simulink model "state_space_all_reduce_uio"  (R2018a)
settings: Solver=FixedStepAuto  StartTime=0.0  StopTime=3  FixedStep=tm  MaxStep=1e-4  RelTol=1e-5  AbsTol=1e-5
InitFcn:
  | SimulinkInit_linea_transmision
values from neighbouring files (symbols this model uses):
  b = 4.91    [SimulinkInit_linea_transmision.m]
  C = 1    [SimulinkInit_linea_transmision.m]
  C1 = 22e-6    (= 2.2e-05)    [SimulinkInit_linea_transmision.m]
  C2 = 22e-6    (= 2.2e-05)    [SimulinkInit_linea_transmision.m]
  C3 = 610e-6    (= 0.00061)    [SimulinkInit_linea_transmision.m]
  Cl = 20000e-6    (= 0.02)    [SimulinkInit_linea_transmision.m]
  Jd = 0.3    [SimulinkInit_linea_transmision.m]
  K = 25    [SimulinkInit_linea_transmision.m]    (also in uio_linear.m = K1+E*H)
  K1 = 9.66    [SimulinkInit_linea_transmision.m]    (also in uio_linear.m = K1')
  K11 = 0.8    [SimulinkInit_linea_transmision.m]
  K1d = 1.15    [SimulinkInit_linea_transmision.m]
  K2 = 6.97    [SimulinkInit_linea_transmision.m]
  K22 = 0.2    [SimulinkInit_linea_transmision.m]
  K2d = 1    [SimulinkInit_linea_transmision.m]
  K3 = 31.8    [SimulinkInit_linea_transmision.m]
  K33 = 0.23    [SimulinkInit_linea_transmision.m]
  K3d = 1    [SimulinkInit_linea_transmision.m]
  K4 = 15.1    [SimulinkInit_linea_transmision.m]
  Kd = 0.02    [SimulinkInit_linea_transmision.m]
  Kdc = 0.02    [SimulinkInit_linea_transmision.m]
  Kf = 1    [SimulinkInit_linea_transmision.m]
  Kh = 1.2    [SimulinkInit_linea_transmision.m]
  Ks = 21.5    [SimulinkInit_linea_transmision.m]
  Ksc = 3    [SimulinkInit_linea_transmision.m]
  Kv = 1    [SimulinkInit_linea_transmision.m]
  L = 5.2    [SimulinkInit_linea_transmision.m]
  L1 = 40e-3    (= 0.04)    [SimulinkInit_linea_transmision.m]
  L2 = 30e-3    (= 0.03)    [SimulinkInit_linea_transmision.m]
  L3 = 5e-3    (= 0.005)    [SimulinkInit_linea_transmision.m]
  L4 = 35e-6    (= 3.5e-05)    [SimulinkInit_linea_transmision.m]
  L5 = 22e-6    (= 2.2e-05)    [SimulinkInit_linea_transmision.m]
  L6 = 10e-6    (= 1e-05)    [SimulinkInit_linea_transmision.m]
  Pd = 0.1    [SimulinkInit_linea_transmision.m]
  R = 10    [SimulinkInit_linea_transmision.m]
  R1 = 0.1    [SimulinkInit_linea_transmision.m]
  R2 = 0.2    [SimulinkInit_linea_transmision.m]
  R3 = 1e-3    (= 0.001)    [SimulinkInit_linea_transmision.m]
  R4 = 0.005    [SimulinkInit_linea_transmision.m]
  R5 = 0.0012    [SimulinkInit_linea_transmision.m]
  R6 = 0.001    [SimulinkInit_linea_transmision.m]
  RL = 10    [SimulinkInit_linea_transmision.m]
  Sbin = 13.8    [SimulinkInit_linea_transmision.m]
  Svin = 2.91    [SimulinkInit_linea_transmision.m]
  T1 = 0.4    [SimulinkInit_linea_transmision.m]
  T2 = 1    [SimulinkInit_linea_transmision.m]
  T3 = 15    [SimulinkInit_linea_transmision.m]
  T4 = 2.5    [SimulinkInit_linea_transmision.m]
  Tao1d = 0.5    [SimulinkInit_linea_transmision.m]
  Tao2d = 0.125    [SimulinkInit_linea_transmision.m]
  Tcd = 0.2    [SimulinkInit_linea_transmision.m]
  Tcr = 0.01    [SimulinkInit_linea_transmision.m]
  Tf = 0.04    [SimulinkInit_linea_transmision.m]
  Tr = 950    [SimulinkInit_linea_transmision.m]
  Tt = 450    [SimulinkInit_linea_transmision.m]
  Ttd = 0.04    [SimulinkInit_linea_transmision.m]
  Tv = 0.05    [SimulinkInit_linea_transmision.m]
  V = 20    [SimulinkInit_linea_transmision.m]
  wref = 70000    [SimulinkInit_linea_transmision.m]
  X_acid = 1.2    [SimulinkInit_linea_transmision.m]
  X_meth = 0.35    [SimulinkInit_linea_transmision.m]
  Z = 3    [SimulinkInit_linea_transmision.m]
undefined symbols (not defined in the file or in its folder): Ad, ataque, Bd, c11, c12, c13, c14, C1o, c21, c22, c23, c24, C2o, c31, c32, c33, c34, C3o, c41, c42, c43, c44, C4o, Cd, F1, F2, F3, F4, H1, H2, H3, H4, K1U, K2U, K3U, K4U, T1s, T2s, T3s, T4s, T5s, tao1, tao2, taod, tm, uio1r, uio2r, uio3r, uio4r
libraries: neural x277, dsparch4 x4, powerlib_meascontrol x4, mpclib x1, simulink x1
(part 1 of 16)
settings Model: Creator=MarioAndres  LastModifiedBy=carma

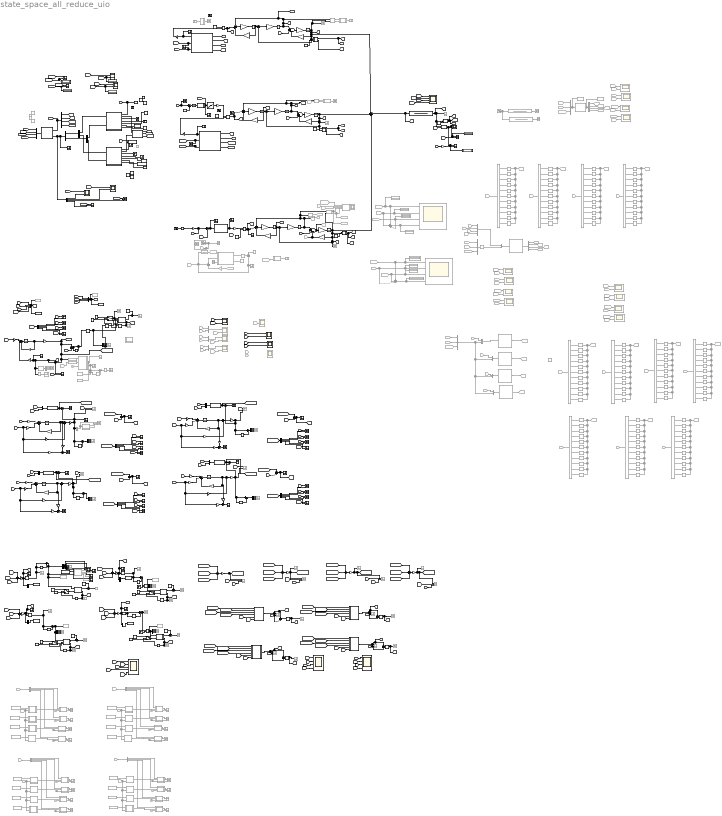
== system state_space_all_reduce_uio ==
  note: Nodo De Optimizacion
  note: CSI1-Biomasa
  note: CSI2-pv
  note: VSI-Diesel
  note: Carga RLC
  note: Attack Detection
  note: Attack Isolation I2
  note: Attack Isolation I3
  note: Attack Isolation I1
  note: Attack Isolation Vsi
  note: Alarm I1
  note: Alarm I3
  note: Alarm I2
  note: Alarm V
  note: Attack Quantification
  1-D Lookup Table2 : Lookup_n-D  NumberOfTableDimensions=1  BreakpointsForDimension1=[0 10 20 30 40 50 70 80 100]  Table=[0 10 200 500 800 1000 1140 1150 1200]  InternalRulePriority=Speed  RndMeth=Simplest  InputSameDT=on
  Abs{,1..3,5..9} (9 alike) : Abs
  Abs4 : Abs  Commented=on
  CSI_Control_BIO : Subsystem  mask{A=[0.0201   -0.039932     0.01986], B=[1     -1.9966       0.998], T=0.0001, st_time=0, Dn=[1     -1.0364], Dd=[1    -0.96364]}
      mask prompts: A "Numerador del control PR(z)"; B "Denominador del control PR(z)"; T "Tiempo de muestreo"; st_time "Tiempo_muerto"; Dn "Dn (Numerador de D(z))"; Dd "Dd (numerador de D(z))"
      mask DialogControl descripcion Prompt: Lazo de control de corriente para inversor monofasico. La entrada es un setpoint de potencia [P, Q]. Con ese setpoint se calcula la referencia de corriente sinusoidal deacuerdo a la tension medida de la red. Por lo anterior este controlador solo es valido para un inversor conectado a la red pues hara que se comporte como un CSI.
      mask DialogControl Control2 Prompt: Dn y Dd corresponden al numerador y denominador de la funcion de transferencia en Z (denominada D(z)) que hara un desfase de 90 de las señales medidas de tension y corriente del inversor. Estos desfases permiten mimificar las señales alfa y beta, de esta forma usar la misma teoria de potencia instantanea para el caso monofasico.
  CSI_Control_BIO1 : Subsystem  mask{A=[0.0201   -0.039932     0.01986], B=[1     -1.9966       0.998], T=0.0001, st_time=0, Dn=[1     -1.0364], Dd=[1    -0.96364]}
      mask prompts: A "Numerador del control PR(z)"; B "Denominador del control PR(z)"; T "Tiempo de muestreo"; st_time "Tiempo_muerto"; Dn "Dn (Numerador de D(z))"; Dd "Dd (numerador de D(z))"
      mask DialogControl descripcion Prompt: Lazo de control de corriente para inversor monofasico. La entrada es un setpoint de potencia [P, Q]. Con ese setpoint se calcula la referencia de corriente sinusoidal deacuerdo a la tension medida de la red. Por lo anterior este controlador solo es valido para un inversor conectado a la red pues hara que se comporte como un CSI.
      mask DialogControl Control2 Prompt: Dn y Dd corresponden al numerador y denominador de la funcion de transferencia en Z (denominada D(z)) que hara un desfase de 90 de las señales medidas de tension y corriente del inversor. Estos desfases permiten mimificar las señales alfa y beta, de esta forma usar la misma teoria de potencia instantanea para el caso monofasico.
  Clock : Clock
  Clock{1,4..19} (17 alike) : Clock  Commented=on
  Clock2 : Clock
  Constant : Constant  Commented=on  Value=-400
  Constant1 : Constant  Commented=on  Value=5000
  Constant{5..6,9..10,12,22..23,27..28,32} (10 alike) : Constant
  Constant{4,11,14,18,20,25} (6 alike) : Constant  Value=1000
  Constant13 : Constant  Value=500
  Constant15 : Constant  Value=1528
  Constant16 : Constant  Value=1200
  Constant17 : Constant  Value=115400
  Constant19 : Constant  Value=800
  Constant2 : Constant  Commented=on  Value=5000
  Constant{7..8,21,24,31} (5 alike) : Constant  Value=0
  Constant26 : Constant  Commented=on  Value=11210
  Constant29 : Constant  Commented=on  Value=1000
  Constant3 : Constant  Commented=on  Value=8000
  Constant30 : Constant  Commented=on  Value=0.1
  Constant{33..36} (4 alike) : Constant  Value=ataque
  Constant37 : Constant  Value=[c11 c12 c13 c14]
  Constant38 : Constant  Commented=on  Value=[c11 c11 c11]
  Constant39 : Constant  Commented=on  Value=[c12 c12 c12]
  Constant40 : Constant  Commented=on  Value=[c13 c13 c13]
  Constant41 : Constant  Commented=on  Value=[c14 c14 c14]
  Constant42 : Constant  Commented=on  Value=[c21 c21 c21]
  Constant43 : Constant  Commented=on  Value=[c22 c22 c22]
  Constant44 : Constant  Commented=on  Value=[c23 c23 c23]
  Constant45 : Constant  Commented=on  Value=[c24 c24 c24]
  Constant46 : Constant  Commented=on  Value=[c31 c31 c31]
  Constant47 : Constant  Commented=on  Value=[c32 c32 c32]
  Constant48 : Constant  Commented=on  Value=[c33 c33 c33]
  Constant49 : Constant  Commented=on  Value=[c34 c34 c34]
  Constant50 : Constant  Commented=on  Value=[c41 c41 c41]
  Constant51 : Constant  Commented=on  Value=[c42 c42 c42]
  Constant52 : Constant  Commented=on  Value=[c43 c43 c43]
  Constant53 : Constant  Commented=on  Value=[c44 c44 c44]  VectorParams1D=off
  Control PR VSI1 : Subsystem
  Current Panel : Constant  Value=1.5
  Delay : Delay  DelayLength=1
  Delay{1..2,16,30,34} (5 alike) : Delay  Commented=on  DelayLength=11
  Delay{10,13,24,27} (4 alike) : Delay  Commented=on  DelayLength=3
  Delay{57,71,85,90,100..101,112} (7 alike) : Delay  Commented=on  DelayLength=8  SampleTime=2*tm
  Delay{46..47,58,62,72,102,113} (7 alike) : Delay  Commented=on  DelayLength=9  SampleTime=2*tm
  Delay{48,59,63,74,91,103,114} (7 alike) : Delay  Commented=on  DelayLength=10  SampleTime=2*tm
  Delay{49,60,64,75,92,104,115} (7 alike) : Delay  Commented=on  DelayLength=11  SampleTime=2*tm
  Delay{50,61,73,76,93,105,116} (7 alike) : Delay  Commented=on  DelayLength=1  SampleTime=2*tm
  Delay{51,65,77..78,94,106,117} (7 alike) : Delay  Commented=on  SampleTime=2*tm
  Delay{52,66,79..80,95,107,118} (7 alike) : Delay  Commented=on  DelayLength=3  SampleTime=2*tm
  Delay{53,67,81,86,96,108,119} (7 alike) : Delay  Commented=on  DelayLength=4  SampleTime=2*tm
  Delay{54,68,82,87,97,109,120} (7 alike) : Delay  Commented=on  DelayLength=5  SampleTime=2*tm
  Delay{11,14,25,28} (4 alike) : Delay  Commented=on
  Delay{55,69,83,88,98,110,121} (7 alike) : Delay  Commented=on  DelayLength=6  SampleTime=2*tm
  Delay{56,70,84,89,99,111,122} (7 alike) : Delay  Commented=on  DelayLength=7  SampleTime=2*tm
  Delay{12,15,26,29} (4 alike) : Delay  Commented=on  DelayLength=1
  Delay{3,17,31,39} (4 alike) : Delay  Commented=on  DelayLength=10
  Delay{4,18,32,40} (4 alike) : Delay  Commented=on  DelayLength=9
  Delay{5,19,33,41} (4 alike) : Delay  Commented=on  DelayLength=8
  Delay{6,20,35,42} (4 alike) : Delay  Commented=on  DelayLength=7
  Delay{7,21,36,43} (4 alike) : Delay  Commented=on  DelayLength=6
  Delay{8,22,37,44} (4 alike) : Delay  Commented=on  DelayLength=5
  Delay{9,23,38,45} (4 alike) : Delay  Commented=on  DelayLength=4
  Demux{,5,7,18..22} (8 alike) : Demux  Commented=on
  Demux{1..4,6,8..17,24,26..29} (20 alike) : Demux
  Derivative1 : Derivative
  Derivative4 : Derivative  Commented=on  CoefficientInTFapproximation=0
  Diesel Generator2 : Subsystem  Commented=on
  Discrete State-Space : DiscreteStateSpace  A=uio1r.A  B=uio1r.B  C=uio1r.C  D=uio1r.D  SampleTime=tm
  Discrete State-Space1 : DiscreteStateSpace  A=uio4r.A  B=uio4r.B  C=uio4r.C  D=uio4r.D  SampleTime=tm
  Discrete State-Space2 : DiscreteStateSpace  A=uio2r.A  B=uio2r.B  C=uio2r.C  D=uio2r.D  SampleTime=tm
  Discrete State-Space3 : DiscreteStateSpace  A=uio3r.A  B=uio3r.B  C=uio3r.C  D=uio3r.D  SampleTime=tm
  Display{,1..3,6..9} (8 alike) : Display  Commented=on
      Display settings: Decimation=6
      Display1 settings: Decimation=3
      Display2 settings: Decimation=3
      Display3 settings: Decimation=6
      Display6 settings: Decimation=2
      Display7 settings: Decimation=3
      Display8 settings: Decimation=3
      Display9 settings: Decimation=2
  Display{4..5,10..13} (6 alike) : Display
      Display10 settings: Decimation=3
      Display11 settings: Decimation=3
      Display12 settings: Decimation=3
      Display13 settings: Decimation=3
      Display4 settings: Decimation=3
      Display5 settings: Decimation=2
  From : From  Commented=on  GotoTag=i1model
  From14 : From  Commented=on  GotoTag=i1
  From{15,47,184,214} (4 alike) : From  Commented=on  GotoTag=i2
  From{24,154,185,215} (4 alike) : From  Commented=on  GotoTag=Vload
  From160 : From  Commented=on  GotoTag=Qo_diesel
  From161 : From  Commented=on  GotoTag=Po_diesel2
  From162 : From  Commented=on  GotoTag=Po_diesel
  From163 : From  Commented=on  GotoTag=Po_bio
  From164 : From  Commented=on  GotoTag=Qo_bio
  From165 : From  Commented=on  GotoTag=Qo_diesel2
  From167 : From  Commented=on  GotoTag=I3
  From168 : From  Commented=on  GotoTag=I2
  From169 : From  Commented=on  GotoTag=I1
  From170 : From  Commented=on  GotoTag=I1r
  From171 : From  Commented=on  GotoTag=I2r
  From172 : From  Commented=on  GotoTag=I3r
  From174 : From  Commented=on  GotoTag=ruo1
  From176 : From  Commented=on  GotoTag=ruo3
  From177 : From  Commented=on  GotoTag=ruo2
  From181 : From  Commented=on  GotoTag=Vlreal
  From182 : From  Commented=on  GotoTag=i1model
  From183 : From  Commented=on  GotoTag=i1
  From186 : From  Commented=on  GotoTag=i3
  From187 : From  Commented=on  GotoTag=i2model
  From188 : From  Commented=on  GotoTag=i3model
  From189 : From  Commented=on  GotoTag=Vloadm
  From190 : From  Commented=on  GotoTag=u2
  From191 : From  Commented=on  GotoTag=u3
  From192 : From  Commented=on  GotoTag=u1
  From193 : From  Commented=on  GotoTag=i1model
  From194 : From  Commented=on  GotoTag=i2model
  From195 : From  Commented=on  GotoTag=i3model
  From196 : From  Commented=on  GotoTag=Vloadm
  From197 : From  Commented=on  GotoTag=i1nn
  From198 : From  Commented=on  GotoTag=i2nn
  From199 : From  Commented=on  GotoTag=i3nn
  From200 : From  Commented=on  GotoTag=vnn
  From201 : From  Commented=on  GotoTag=u2nn
  From202 : From  Commented=on  GotoTag=u3nn
  From203 : From  Commented=on  GotoTag=u1nn
  From204 : From  Commented=on  GotoTag=i1model1
  From205 : From  Commented=on  GotoTag=i2model1
  From206 : From  Commented=on  GotoTag=i3model1
  From207 : From  Commented=on  GotoTag=Vloadm1
  From208 : From  Commented=on  GotoTag=i1nn1
  From209 : From  Commented=on  GotoTag=i2nn1
  From210 : From  Commented=on  GotoTag=i3nn1
  From211 : From  Commented=on  GotoTag=vnn1
  From212 : From  Commented=on  GotoTag=i1model1
  From213 : From  Commented=on  GotoTag=i1
  From216 : From  Commented=on  GotoTag=i3
  From217 : From  Commented=on  GotoTag=i2model1
  From218 : From  Commented=on  GotoTag=i3model1
  From219 : From  Commented=on  GotoTag=Vloadm1
  From220 : From  Commented=on  GotoTag=u1
  From221 : From  Commented=on  GotoTag=u2
  From222 : From  Commented=on  GotoTag=u3
  From{224,226,228,230} (4 alike) : From  Commented=on  GotoTag=u_fs
  From225 : From  Commented=on  GotoTag=uio1
  From227 : From  Commented=on  GotoTag=uio2
  From229 : From  Commented=on  GotoTag=uio3
  From231 : From  Commented=on  GotoTag=uio4
  From25 : From  Commented=on  GotoTag=i3
  From264 : From  Commented=on  GotoTag=I3
  From269 : From  Commented=on  GotoTag=I3r
  From30 : From  Commented=on  GotoTag=u2
  From33 : From  Commented=on  GotoTag=u3
  From37 : From  Commented=on  GotoTag=Papadiel
  From38 : From  Commented=on  GotoTag=Paparente
  From39 : From  Commented=on  GotoTag=Q_ref
  From40 : From  Commented=on  GotoTag=P_ref
  From41 : From  Commented=on  GotoTag=Io_diesel
  From6 : From  Commented=on  GotoTag=i2model
  From60 : From  Commented=on  GotoTag=y_ma
  From7 : From  Commented=on  GotoTag=i3model
  From8 : From  Commented=on  GotoTag=Vloadm
  From9 : From  Commented=on  GotoTag=u1
  Function Fitting Neural Network : Subsystem  Commented=on
      mask help: Function Fitting Neural Network
      mask Display: e = 0.06;c1 = [120 150 230]/255;c2 = ([120 150 230]+0)/383;c3 = ([120 150 230]+128)/383;patch([0 1 1 0],[0 0 1 1],c1);patch([0 1 1 1-e 1-e 0+e],[0 0 1 1-e 0+e 0+e],c2);patch([0 0 1 1-e 0+e 0+e],[0 1 1 1-e 1-e 0+e],c3);plot([0 1 1 0 0],[0 0 1 1 0]);fprintf('NNET');port_label('input',1,' Input');port_label('output',1,'Output ');
  Function Fitting Neural Network1 : Subsystem  Commented=on
      mask help: Function Fitting Neural Network
      mask Display: e = 0.06;c1 = [120 150 230]/255;c2 = ([120 150 230]+0)/383;c3 = ([120 150 230]+128)/383;patch([0 1 1 0],[0 0 1 1],c1);patch([0 1 1 1-e 1-e 0+e],[0 0 1 1-e 0+e 0+e],c2);patch([0 0 1 1-e 0+e 0+e],[0 1 1 1-e 1-e 0+e],c3);plot([0 1 1 0 0],[0 0 1 1 0]);fprintf('NNET');port_label('input',1,' Input');port_label('output',1,'Output ');
  Function Fitting Neural Network2 : Subsystem  Commented=on
      mask help: Function Fitting Neural Network
      mask Display: e = 0.06;c1 = [120 150 230]/255;c2 = ([120 150 230]+0)/383;c3 = ([120 150 230]+128)/383;patch([0 1 1 0],[0 0 1 1],c1);patch([0 1 1 1-e 1-e 0+e],[0 0 1 1-e 0+e 0+e],c2);patch([0 0 1 1-e 0+e 0+e],[0 1 1 1-e 1-e 0+e],c3);plot([0 1 1 0 0],[0 0 1 1 0]);fprintf('NNET');port_label('input',1,' Input');port_label('output',1,'Output ');
  Function Fitting Neural Network3 : Subsystem  Commented=on
      mask help: Function Fitting Neural Network
      mask Display: e = 0.06;c1 = [120 150 230]/255;c2 = ([120 150 230]+0)/383;c3 = ([120 150 230]+128)/383;patch([0 1 1 0],[0 0 1 1],c1);patch([0 1 1 1-e 1-e 0+e],[0 0 1 1-e 0+e 0+e],c2);patch([0 0 1 1-e 0+e 0+e],[0 1 1 1-e 1-e 0+e],c3);plot([0 1 1 0 0],[0 0 1 1 0]);fprintf('NNET');port_label('input',1,' Input');port_label('output',1,'Output ');
  Function Fitting Neural Network4 : Subsystem  Commented=on
      mask help: Function Fitting Neural Network
      mask Display: e = 0.06;c1 = [120 150 230]/255;c2 = ([120 150 230]+0)/383;c3 = ([120 150 230]+128)/383;patch([0 1 1 0],[0 0 1 1],c1);patch([0 1 1 1-e 1-e 0+e],[0 0 1 1-e 0+e 0+e],c2);patch([0 0 1 1-e 0+e 0+e],[0 1 1 1-e 1-e 0+e],c3);plot([0 1 1 0 0],[0 0 1 1 0]);fprintf('NNET');port_label('input',1,' Input');port_label('output',1,'Output ');
  Gain : Gain  Gain=1/L1
  Gain1 : Gain  Gain=1/C1
  Gain10 : Gain  Gain=1/L3
  Gain11 : Gain  Gain=1/C3
  Gain12 : Gain  Gain=1/L6
  Gain13 : Gain  Gain=R6
  Gain14 : Gain  Gain=R3
  Gain{15..18} (4 alike) : Gain  Gain=2
  Gain2 : Gain  Gain=1/L4
  Gain20 : Gain  Gain=-1
  Gain21 : Gain  Commented=on  Gain=.5
  Gain{22..29} (8 alike) : Gain  Gain=1/3
  Gain3 : Gain  Gain=R4
  Gain30 : Gain  Gain=C3
  Gain4 : Gain  Gain=R1
  Gain5 : Gain  Gain=1/L2
  Gain6 : Gain  Gain=1/C2
  Gain7 : Gain  Gain=1/L5
  Gain8 : Gain  Gain=R5
  Gain9 : Gain  Gain=R2
  Goto : Goto  Commented=on  GotoTag=i1model
  Goto15 : Goto  Commented=on  GotoTag=i2model
  Goto16 : Goto  Commented=on  GotoTag=i3model
  Goto17 : Goto  Commented=on  GotoTag=v3
  Goto18 : Goto  Commented=on  GotoTag=vl6
  Goto19 : Goto  Commented=on  GotoTag=vr6
  Goto22 : Goto  Commented=on  GotoTag=Vloadm
  Goto23 : Goto  Commented=on  GotoTag=Vdc
  Goto24 : Goto  Commented=on  GotoTag=Io_diesel
  Goto61 : Goto  Commented=on  GotoTag=V_vsi
  Goto62 : Goto  Commented=on  GotoTag=a4
  Goto74 : Goto  Commented=on  GotoTag=Qo_diesel2
  Goto75 : Goto  Commented=on  GotoTag=Po_diesel2
  Goto79 : Goto  Commented=on  GotoTag=i1model
  Goto80 : Goto  Commented=on  GotoTag=i2model
  Goto81 : Goto  Commented=on  GotoTag=i3model
  Goto82 : Goto  Commented=on  GotoTag=Vloadm
  Goto83 : Goto  Commented=on  GotoTag=i1nn
  Goto84 : Goto  Commented=on  GotoTag=i2nn
  Goto85 : Goto  Commented=on  GotoTag=i3nn
  Goto86 : Goto  Commented=on  GotoTag=vnn
  Goto87 : Goto  Commented=on  GotoTag=i1model1
  Goto88 : Goto  Commented=on  GotoTag=i2model1
  Goto89 : Goto  Commented=on  GotoTag=i3model1
  Goto90 : Goto  Commented=on  GotoTag=Vloadm1
  Goto91 : Goto  Commented=on  GotoTag=i1nn1
  Goto92 : Goto  Commented=on  GotoTag=i2nn1
  Goto93 : Goto  Commented=on  GotoTag=i3nn1
  Goto94 : Goto  Commented=on  GotoTag=vnn1
  Goto95 : Goto  Commented=on  GotoTag=u1nn
  Goto96 : Goto  Commented=on  GotoTag=u2nn
  Goto97 : Goto  Commented=on  GotoTag=u3nn
  Integrator{,1..8} (9 alike) : Integrator
  Integrator9 : Integrator  LimitOutput=on  UpperSaturationLimit=1  LowerSaturationLimit=0
  LinearProg2 : MATLAB Function  TreatAsAtomicUnit=on  SystemSampleTime=1e-3
  LinearProg3 : MATLAB Function  TreatAsAtomicUnit=on  SystemSampleTime=1e-3
  MATLAB Funcionando sin Vload conectado despues del ataque : MATLAB Function  Commented=on  TreatAsAtomicUnit=on
  MATLAB Function : MATLAB Function  Commented=on  TreatAsAtomicUnit=on
  "MATLAB Function SOC " : MATLAB Function  TreatAsAtomicUnit=on
  MATLAB Function1 : MATLAB Function  TreatAsAtomicUnit=on
  MATLAB Function10 : MATLAB Function  Commented=on  TreatAsAtomicUnit=on
  MATLAB Function11 : MATLAB Function  Commented=on  TreatAsAtomicUnit=on
  MATLAB Function12 : MATLAB Function  TreatAsAtomicUnit=on
  MATLAB Function13 : MATLAB Function  TreatAsAtomicUnit=on
  MATLAB Function14 : MATLAB Function  Commented=on  TreatAsAtomicUnit=on
  MATLAB Function15 : MATLAB Function  Commented=on  TreatAsAtomicUnit=on
  MATLAB Function16 : MATLAB Function  Commented=on  TreatAsAtomicUnit=on
  MATLAB Function17 : MATLAB Function  TreatAsAtomicUnit=on
  MATLAB Function18 : MATLAB Function  TreatAsAtomicUnit=on
  MATLAB Function19 : MATLAB Function  Commented=on  TreatAsAtomicUnit=on
  MATLAB Function2 : MATLAB Function  TreatAsAtomicUnit=on
  MATLAB Function20 : MATLAB Function  Commented=on  TreatAsAtomicUnit=on
  MATLAB Function21 : MATLAB Function  Commented=on  TreatAsAtomicUnit=on
  MATLAB Function22 : MATLAB Function  Commented=on  TreatAsAtomicUnit=on
  MATLAB Function23 : MATLAB Function  Commented=on  TreatAsAtomicUnit=on
  MATLAB Function24 : MATLAB Function  Commented=on  TreatAsAtomicUnit=on
  MATLAB Function25 : MATLAB Function  Commented=on  TreatAsAtomicUnit=on
  MATLAB Function26 : MATLAB Function  Commented=on  TreatAsAtomicUnit=on
  MATLAB Function27 : MATLAB Function  Commented=on  TreatAsAtomicUnit=on
  MATLAB Function28 : MATLAB Function  Commented=on  TreatAsAtomicUnit=on
  MATLAB Function29 : MATLAB Function  Commented=on  TreatAsAtomicUnit=on
  MATLAB Function3 : MATLAB Function  Commented=on  TreatAsAtomicUnit=on
  MATLAB Function34 : MATLAB Function  TreatAsAtomicUnit=on
  MATLAB Function36 : MATLAB Function  TreatAsAtomicUnit=on
  MATLAB Function38 : MATLAB Function  TreatAsAtomicUnit=on
  MATLAB Function39 : MATLAB Function  TreatAsAtomicUnit=on
  MATLAB Function4 : MATLAB Function  Commented=on  TreatAsAtomicUnit=on
  MATLAB Function5 : MATLAB Function  Commented=on  TreatAsAtomicUnit=on
  MATLAB Function6 : MATLAB Function  Commented=on  TreatAsAtomicUnit=on
  MATLAB Function7 : MATLAB Function  Commented=on  TreatAsAtomicUnit=on
  MATLAB Function8 : MATLAB Function  Commented=on  TreatAsAtomicUnit=on
  MPC Controller : mpclib/MPC Controller  SCDEnableBlockLinearizationSpecification=on  mpcobj=mpcobj  is_multiple=0  enable_value=0  return_u0=off  updateMPCinCallerWorkspace=on  ref_from_ws=off  ref_signal_name=[]  ref_preview=off  md_from_ws=off  md_signal_name=[]  md_preview=off  from_project=off  project_file=MPCtask.mat  md_inport=off  mv_inport=off  cost_outport=off  return_sequence=off  return_qpstatus=off  return_state=off  state_inport=off  lims_inport=off  cc_inport=off  ywt_inport=off  is_designfromscratch=0  uwt_inport=off  duwt_inport=off  rhoeps_inport=off  uref_inport=off  n_ts=0.1  n_p=100  n_mv=4  n_md=0  n_ud=0  n_mo=4  n_uo=0  BlockDataType=double  SampleTimeInherited=off  switch_inport=off
  MeasureNode_I1 : Subsystem
  MeasureNode_I2 : Subsystem
  MeasureNode_I3 : Subsystem
  MeasureNode_I4 : Subsystem
  MeasureNode_I5 : Subsystem  Commented=on
  Memory{,1..13} (14 alike) : Memory
  Memory14 : Memory  Commented=on
  Mux{,14,16..18,26..28} (8 alike) : Mux  Commented=on  Inputs=2
  Mux1 : Mux  Commented=on  Inputs=3
  Mux{9..12,19..25} (11 alike) : Mux  Commented=on  Inputs=11
  Mux13 : Mux  Commented=on
  Mux15 : Mux  Commented=on  Inputs=3
  Mux2 : Mux  Commented=on  Inputs=3
  Mux{3,5..6,29..32} (7 alike) : Mux  Inputs=2
  Mux4 : Mux
  Mux7 : Mux  Inputs=3
  Mux8 : Mux
  PID Controller2 : simulink/Continuous/PID Controller  Commented=on  Controller=PID  TimeDomain=Continuous-time  SampleTime=-1  IntegratorMethod=Forward Euler  FilterMethod=Forward Euler  Form=Parallel  UseFilter=on  ControllerParametersSource=internal  P=0.000853612192208084  I=3.94394231511782e-05  D=0.00224356290205903  N=0.155980576752107  InitialConditionSource=internal  InitialConditionForIntegrator=0  InitialConditionForFilter=0  ExternalReset=none  LimitOutput=off  UpperSaturationLimit=inf  LowerSaturationLimit=-inf  LinearizeAsGain=on  AntiWindupMode=none  Kb=1  TrackingMode=off  Kt=1  PParamMin=[]  PParamMax=[]  IParamMin=[]  IParamMax=[]  DParamMin=[]  DParamMax=[]  NParamMin=[]  NParamMax=[]  KbParamMin=[]  KbParamMax=[]  KtParamMin=[]  KtParamMax=[]  POutMin=[]  POutMax=[]  IOutMin=[]  IOutMax=[]  DOutMin=[]  DOutMax=[]  NOutMin=[]  NOutMax=[]  KbOutMin=[]  KbOutMax=[]  KtOutMin=[]  KtOutMax=[]  IntegratorOutMin=[]  IntegratorOutMax=[]  FilterOutMin=[]  FilterOutMax=[]  SumOutMin=[]  SumOutMax=[]  SumI1OutMin=[]  SumI1OutMax=[]  SumI2OutMin=[]  SumI2OutMax=[]  SumI3OutMin=[]  SumI3OutMax=[]  SumDOutMin=[]  SumDOutMax=[]  SaturationOutMin=[]  SaturationOutMax=[]  IntegratorContinuousStateAttributes=''  IntegratorStateMustResolveToSignalObject=off  IntegratorRTWStateStorageClass=Auto  FilterContinuousStateAttributes=''  FilterStateMustResolveToSignalObject=off  FilterRTWStateStorageClass=Auto  DifferentiatorICPrevScaledInput=0  DifferentiatorOutMin=[]  DifferentiatorOutMax=[]  InitialConditionSetting=State (most efficient)  FilterDiffOutCoefMin=[]  FilterDiffOutCoefMax=[]  SumDenOutMin=[]  SumDenOutMax=[]  SumNumOutMin=[]  SumNumOutMax=[]  ReciprocalOutMin=[]  ReciprocalOutMax=[]  DivideOutMin=[]  DivideOutMax=[]  TunerSelectOption=Transfer Function Based (PID Tuner App)
  Power : powerlib_meascontrol/Measurements/Power  Freq=60  Vinit=[1, 0]  Iinit=[1, 0]  Ts=0
      settings: SourceProductName=Simscape Power Systems
  Power1 : powerlib_meascontrol/Measurements/Power  Commented=on  Freq=60  Vinit=[1, 0]  Iinit=[1, 0]  Ts=0
      settings: SourceProductName=Simscape Power Systems
  Power3 : powerlib_meascontrol/Measurements/Power  Commented=on  Freq=60  Vinit=[1, 0]  Iinit=[1, 0]  Ts=0
      settings: SourceProductName=Simscape Power Systems
  Power4 : powerlib_meascontrol/Measurements/Power  Commented=on  Freq=60  Vinit=[1, 0]  Iinit=[1, 0]  Ts=0
      settings: SourceProductName=Simscape Power Systems
  Product{,1..4} (5 alike) : Product
  Random Number : RandomNumber  Mean=1500  Variance=1500000  SampleTime=0.5
  Random Number1 : RandomNumber  Mean=1000  Variance=1500000  SampleTime=0.5
  Random Number2 : RandomNumber  Mean=1000  Variance=1500000  SampleTime=0.5
  Random Number3 : RandomNumber  Mean=1200  Variance=1500000  SampleTime=0.5
  Random Number4 : RandomNumber  Mean=500  Variance=1500  SampleTime=0.5
  Random Number5 : RandomNumber  Mean=800  Variance=1500  SampleTime=0.5
  Scope{,1,3,7,35,52..53,58,74,86..90,95,97,104..109,111,113,115..116,123..134,136..137,140,169} (42 alike) : Scope  Commented=on  NumInputPorts=2
  Scope{8,10..12,14..18,21,98..102,119,122,141..146,151..168} (41 alike) : Scope  NumInputPorts=2
  Scope{2,4..6,9,22,24..25,31,34,36..42,46..47,49..51,55..57,64,68..71,73,75,91,94,96,103,120..121,135,139} (40 alike) : Scope  Commented=on
  Scope{13,19..20,26..30,32,43..45,48,61,65..67,72,110,112,114,118,147..150} (26 alike) : Scope
  Scope{59..60,62,117,138} (5 alike) : Scope  Commented=on  NumInputPorts=3
  Scope23 : Scope  NumInputPorts=4
  Scope{33,54,76..83,92..93} (12 alike) : Scope  Commented=on  NumInputPorts=4
  Scope63 : Scope  NumInputPorts=4
  Scope84 : Scope  NumInputPorts=5
  Scope85 : Scope  NumInputPorts=4
  Signal Specification : SignalSpecification  Commented=on  Dimensions=4
  Signal Specification1 : SignalSpecification  Commented=on  Dimensions=4
  Sine Wave : Sin  Commented=on  Amplitude=128  Frequency=2*pi*60  SampleTime=0
  Sine Wave2 : Sin  Frequency=2*pi/0.025  SampleTime=0
  Sine Wave3 : Sin  Frequency=2*pi/0.025  SampleTime=0
  Sine Wave4 : Sin  Commented=on  Amplitude=170  Frequency=2*pi*60  SampleTime=0
  Sine Wave5 : Sin  Amplitude=60  Frequency=2*pi*60  SampleTime=0
  Sine Wave6 : Sin  Amplitude=211  Frequency=2*pi*60  SampleTime=0
  State-Space : StateSpace  Commented=on  A=|  B=|  C=[zeros(1,3) 1 zeros(1,7); zeros(1,4) 1 zeros(1,6); zeros(1,5) 1 zeros(1,5);zeros(1,10) 1]  D=zeros(4,3);  InitialCondition=0
      A=|
      | [-R1/L1 zeros(1,6) -1/L1 zeros(1,3);
      |     0 -R2/L2 zeros(1,6) -1/L2 0 0;
      |     zeros(1,2) -R3/L3 zeros(1,6) -1/L3 0;
      |     zeros(1,3) -R4/L4 zeros(1,3) 1/L4 0 0 -1/L4;
      |     zeros(1,4) -R5/L5 zeros(1,3) 1/L5 0 -1/L5;
      |     zeros(1,5) -R6/L6 zeros(1,3) 1/L6 -1/L6;
      |     zeros(1,6) -R/L zeros(1,3) 1/L;
      |     1/C1 zeros(1,2) -1/C1 zeros(1,7);
      |     0 1/C2 0 0 -1/C2 zeros(1,6);
      |     0 0 1/C3 0 0 -1/C3 zeros(1,5);
      |     zeros(1,3) 1/Cl 1/Cl 1/Cl -1/Cl zeros(1,3) -1/(Cl*RL)]
      B=|
      | [1/L1 0 0;
      |    0 1/L2 0;
      |    0 0 1/L3;
      |    zeros(8,3)];
  Step : Step  Commented=on  Time=0  After=28  SampleTime=0
  Step1 : Step  Time=200  Before=1.2  After=.4  SampleTime=0
  Step10 : Step  Time=20  Before=115400  After=15400  SampleTime=0
  Step13 : Step  Time=0.1  SampleTime=0
  Step14 : Step  Time=0.1  SampleTime=0
  Step4 : Step  Time=200  Before=1.2  After=0.4  SampleTime=0
  Step5 : Step  Time=200  Before=1  SampleTime=0
  Step8 : Step  Time=200  Before=1  SampleTime=0
  Step9 : Step  Time=20  Before=978  After=1400  SampleTime=0
  Sum{,4,7,17,20,24..26,30,36..37,39..40,44,46..48,50} (18 alike) : Sum  Inputs=|+-
  Sum1 : Sum  Inputs=|+--
  Sum{10,14,22,38,45,74} (6 alike) : Sum  Inputs=|++
  Sum11 : Sum  Commented=on  Inputs=3
  Sum12 : Sum  Commented=on  Inputs=3
  Sum13 : Sum  Commented=on  Inputs=+-
  Sum15 : Sum  Commented=on  Inputs=+-
  Sum{16,18,27,33,42,67,70,72..73} (9 alike) : Sum  Inputs=+-
  Sum{19,31..32,71} (4 alike) : Sum  Inputs=-+|
  Sum2 : Sum  Inputs=|+++
  Sum{21,23,49,75..76} (5 alike) : Sum  Inputs=|+++  SampleTime=tm
  Sum{28..29,34..35,53} (5 alike) : Sum  Inputs=+-|
  Sum3 : Sum  Inputs=-|+-
  Sum41 : Sum  Commented=on  Inputs=|+-
  Sum43 : Sum  Commented=on  Inputs=|+-
  Sum5 : Sum  Inputs=|+--
  Sum{58..61,77..80} (8 alike) : Sum  Inputs=+++
  Sum6 : Sum  Inputs=-|+-
  Sum8 : Sum  Inputs=|+--
  Sum9 : Sum  Inputs=-|+-
  Switch{,1..4} (5 alike) : Switch  Criteria=u2 > Threshold
  To Workspace : ToWorkspace  Commented=on  VariableName=det1  SampleTime=1e-4
  To Workspace1 : ToWorkspace  Commented=on  VariableName=norm1  SampleTime=1e-4
  To Workspace10 : ToWorkspace  VariableName=y4  SampleTime=tm
      settings: Decimation=2
  To Workspace11 : ToWorkspace  Commented=on  VariableName=umbral1  SampleTime=tm
      settings: Decimation=2
  To Workspace12 : ToWorkspace  Commented=on  VariableName=umbral2  SampleTime=tm
      settings: Decimation=2
  To Workspace13 : ToWorkspace  Commented=on  VariableName=umbral3  SampleTime=tm
      settings: Decimation=2
  To Workspace14 : ToWorkspace  Commented=on  VariableName=umbral4  SampleTime=tm
      settings: Decimation=2
  To Workspace15 : ToWorkspace  VariableName=u  SampleTime=tm
      settings: Decimation=2
  To Workspace2 : ToWorkspace  Commented=on  VariableName=y_ma  SampleTime=1e-4
  To Workspace3 : ToWorkspace  Commented=on  VariableName=u_fs  SampleTime=1e-4
  To Workspace4 : ToWorkspace  Commented=on  VariableName=u  SampleTime=tm
      settings: Decimation=2
  To Workspace5 : ToWorkspace  Commented=on  VariableName=y  SampleTime=tm
      settings: Decimation=2
  To Workspace6 : ToWorkspace  VariableName=y_ma  SampleTime=tm
      settings: Decimation=2
  To Workspace7 : ToWorkspace  VariableName=y1  SampleTime=tm
      settings: Decimation=2
  To Workspace8 : ToWorkspace  VariableName=y3  SampleTime=tm
      settings: Decimation=2
  To Workspace9 : ToWorkspace  VariableName=y2  SampleTime=tm
      settings: Decimation=2
  Transfer Fcn2 : TransferFcn  Commented=on  Numerator=[RL*L RL*R]  Denominator="[Cl*RL*L  (R*RL*Cl+L) RL+R]"
  Transfer Fcn3 : TransferFcn  Numerator=[RL*L RL*R]  Denominator="[Cl*RL*L  (R*RL*Cl+L) RL+R]"
  Transfer Fcn4 : TransferFcn  Commented=on  Denominator=[1e-4 1]
  Transfer Fcn5 : TransferFcn  Commented=on  Numerator=[R*RL*L 0]  Denominator=[Cl*RL*R*L (RL+R)*L R*RL]
  Umbral adaptativo1 : Subsystem  Commented=on
  Umbral adaptativo10 : Subsystem  Commented=on
  Umbral adaptativo11 : Subsystem  Commented=on
  Umbral adaptativo12 : Subsystem  Commented=on
  Umbral adaptativo13 : Subsystem  Commented=on
  Umbral adaptativo14 : Subsystem  Commented=on
  Umbral adaptativo15 : Subsystem  Commented=on
  Umbral adaptativo16 : Subsystem  Commented=on
  Umbral adaptativo17 : Subsystem  Commented=on
  Umbral adaptativo2 : Subsystem  Commented=on
  Umbral adaptativo3 : Subsystem  Commented=on
  Umbral adaptativo4 : Subsystem  Commented=on
  Umbral adaptativo5 : Subsystem  Commented=on
  Umbral adaptativo6 : Subsystem  Commented=on
  Umbral adaptativo7 : Subsystem  Commented=on
  Umbral adaptativo8 : Subsystem  Commented=on
  Umbral adaptativo9 : Subsystem  Commented=on
  Unit Delay : UnitDelay  Commented=on  SampleTime=2*tm
  Unit Delay{1..2,6..7,10} (5 alike) : UnitDelay  SampleTime=tm
  adis1 : Gain  Gain=F3  Multiplication=Matrix(K*u) (u vector)  SampleTime=tm
  adis10 : Gain  Gain=Ld'  Multiplication=Matrix(K*u) (u vector)  SampleTime=tm
  adis11 : Gain  Gain=F1  Multiplication=Matrix(K*u) (u vector)  SampleTime=tm
  adis12 : Gain  Gain=F2  Multiplication=Matrix(K*u) (u vector)  SampleTime=tm
  adis2 : Gain  Gain=F4  Multiplication=Matrix(K*u) (u vector)  SampleTime=tm
  adis7 : Gain  Gain=Ad  Multiplication=Matrix(K*u) (u vector)  SampleTime=tm
  bdis1 : Gain  Gain=T3*Bd  Multiplication=Matrix(K*u) (u vector)  SampleTime=tm
  bdis10 : Gain  Gain=T2*Bd  Multiplication=Matrix(K*u) (u vector)  SampleTime=tm
  bdis11 : Gain  Gain=K2U  Multiplication=Matrix(K*u) (u vector)  SampleTime=tm
  bdis12 : Gain  Gain=H2  Multiplication=Matrix(K*u) (u vector)  SampleTime=tm
  bdis13 : Gain  Gain=eye(1)-C2o*H2  Multiplication=Matrix(K*u) (u vector)  SampleTime=tm
  bdis14 : Gain  Gain=eye(1)-C1o*H1  Multiplication=Matrix(K*u) (u vector)  SampleTime=tm
  bdis15 : Gain  Gain=C1o  Multiplication=Matrix(K*u) (u vector)  SampleTime=tm
  bdis16 : Gain  Gain=C2o  Multiplication=Matrix(K*u) (u vector)  SampleTime=tm
  bdis17 : Gain  Gain=T4*Bd  Multiplication=Matrix(K*u) (u vector)  SampleTime=tm
  bdis18 : Gain  Gain=K4U  Multiplication=Matrix(K*u) (u vector)  SampleTime=tm
  bdis19 : Gain  Gain=H4  Multiplication=Matrix(K*u) (u vector)  SampleTime=tm
  bdis2 : Gain  Gain=K3U  Multiplication=Matrix(K*u) (u vector)  SampleTime=tm
  bdis20 : Gain  Gain=eye(1)-C4o*H4  Multiplication=Matrix(K*u) (u vector)  SampleTime=tm
  bdis21 : Gain  Gain=C4o  Multiplication=Matrix(K*u) (u vector)  SampleTime=tm
  bdis3 : Gain  Gain=H3  Multiplication=Matrix(K*u) (u vector)  SampleTime=tm
  bdis4 : Gain  Gain=eye(1)-C3o*H3  Multiplication=Matrix(K*u) (u vector)  SampleTime=tm
  bdis5 : Gain  Gain=Bd  Multiplication=Matrix(K*u) (u vector)  SampleTime=tm
  bdis6 : Gain  Gain=C3o  Multiplication=Matrix(K*u) (u vector)  SampleTime=tm
  bdis7 : Gain  Gain=T1*Bd  Multiplication=Matrix(K*u) (u vector)  SampleTime=tm
  bdis8 : Gain  Gain=K1U  Multiplication=Matrix(K*u) (u vector)  SampleTime=tm
  bdis9 : Gain  Gain=H1  Multiplication=Matrix(K*u) (u vector)  SampleTime=tm
  cdis{1..5} (5 alike) : Gain  Gain=Cd  Multiplication=Matrix(K*u) (u vector)  SampleTime=tm
  generador biomasa : Subsystem  Commented=on
  wires:
  Gain/1 -> Integrator/1
  Integrator/1 -> Gain4/1, Sum/1
  Sum/1 -> Gain1/1
  Gain1/1 -> Integrator1/1
  Integrator1/1 -> [v1], [V_bio], Sum3/1, Power3/1, Sum1/1
  Sum1/1 -> Gain2/1
  Gain2/1 -> Integrator2/1
  Integrator2/1 -> Power3/2, Scope4/1, [I1r], Sum2/1, MeasureNode_I2/1(in), Sum/2, Gain3/1
  Gain3/1 -> Sum1/3
  Sum3/1 -> Gain/1
  Gain4/1 -> Sum3/3
  Sum2/1 -> [I_load], Transfer Fcn3/1
  Transfer Fcn3/1 -> [Vlreal], MeasureNode_I4/1(in), Power/1, Scope2/1
  [Vload] -> Sum1/2
  Integrator3/1 -> [ipi], Gain9/1, Sum4/1
  Gain5/1 -> Integrator3/1
  Gain6/1 -> Integrator4/1
  Gain8/1 -> Sum5/3
  Gain7/1 -> Integrator5/1
  [Vload] -> Sum5/2
  Gain9/1 -> Sum6/3
  Sum6/1 -> Gain5/1
  Sum5/1 -> Gain7/1
  Sum4/1 -> Gain6/1
  Integrator6/1 -> [i3m], Gain14/1, Sum7/1
  Gain10/1 -> Integrator6/1
  Gain11/1 -> Integrator7/1
  Integrator7/1 -> MeasureNode_I5/1(in), Power1/1, Sum9/1, Goto17/1, Sum8/1
  Gain13/1 -> Goto19/1, Sum8/3
  Gain12/1 -> Integrator8/1
  [Vload] -> Sum8/2
  Gain14/1 -> Sum9/3
  Sum9/1 -> Gain10/1
  Sum8/1 -> Goto18/1, Gain12/1
  Sum7/1 -> Gain11/1
  Integrator8/1 -> Power1/2, Sum2/3, MeasureNode_I3/1(in), [I3r], Scope6/1, Sum7/2, Gain13/1
  Integrator5/1 -> Sum2/2, [I2r], Scope5/1, MeasureNode_I1/1(in), Sum4/2, Gain8/1
  [I_load] -> Power/2
  Power/2 -> Display5/1, Scope12/1, Scope10/2
  [P_ref] -> Scope11/2
  CSI_Control_BIO/2(Q_measure) -> [Qo_bio], Scope14/1
  CSI_Control_BIO/3(P_measure) -> [Po_bio], Scope14/2
  Control PR VSI1/1(d) -> Gain17/1, Scope28/1
  Product3/1 -> [u3], Sum9/2, Scope29/1
  CSI_Control_BIO1/2(Q_measure) -> [Qo_diesel], Scope21/1
  CSI_Control_BIO1/3(P_measure) -> [Po_diesel], Scope21/2
  Integrator4/1 -> [v2], [V_die], Power4/1, Sum6/1, Sum5/1
  Current Panel/1 -> Sum14/2
  Sum14/1 -> Integrator9/1
  [ipi] -> Scope27/1, Sum14/1  "inductor I measured"
  "MATLAB Function SOC "/1(y) -> [SOC], Scope26/1, 1-D Lookup Table2/1  "soc"
  1-D Lookup Table2/1 -> Gain18/1  "battery Vdc"
  Integrator9/1 -> "MATLAB Function SOC "/1(u)
  Sum44/1 -> Control PR VSI1/1(Ierror), Scope19/1
  Product1/1 -> Sum6/2, [u2]
  Step5/1 -> LinearProg3/3(kb)
  Mux4/1 -> [Paparente], MPC Controller/1
  [Qo_bio] -> Mux4/2
  LinearProg2/2(Pdo) -> Mux6/1  "die"
  Mux6/1 -> Mux3/2
  [SOC] -> MATLAB Function2/1(SOC)
  MPC Controller/1 -> Demux3/1
  [Qo_diesel] -> Mux4/4
  Mux5/1 -> Mux3/1
  [Po_diesel] -> Mux4/3
  Step4/1 -> LinearProg2/4(kd)
  Step1/1 -> LinearProg2/3(kb)
  MATLAB Function2/1(MaxP) -> LinearProg2/2(P_e_alt)
  MATLAB Function2/2(MaxQ) -> LinearProg3/2(Q_e_alt)
  Step8/1 -> LinearProg3/4(kd)
  LinearProg3/2(Qdo) -> Mux6/2
  [Po_bio] -> Mux4/1
  LinearProg3/1(Qbo) -> Mux5/2
  LinearProg2/1(Pbo) -> Mux5/1  "bio"
  [Pi_bio] -> Display12/1, Scope16/2
  [Po_bio] -> Scope16/1
  [Qi_bio] -> Display13/1, Scope15/2
  [Qo_bio] -> Scope15/1
  [Qo_diesel] -> Scope17/1
  [Po_diesel] -> Scope18/1
  [Pi_Diesel] -> Display11/1, Scope18/2
  [V_vsi] -> Scope23/4
  [V_die] -> Scope23/3
  [V_bio] -> Scope23/2
  [Vload] -> Scope23/1
  generador biomasa/1(Vdc) -> Scope24/1
  Step/1 -> generador biomasa/1(In1)
  [v2] -> CSI_Control_BIO1/1(V_measured)
  [i2] -> CSI_Control_BIO1/2(I_measured)
  [v1] -> CSI_Control_BIO/1(V_measured)
  [i1] -> CSI_Control_BIO/2(I_measured)
  Gain18/1 -> Product1/1
  Gain15/1 -> Product/2
  Product/1 -> [u1], Sum3/2
  Gain16/1 -> Product1/2
  [Pi_Diesel] -> CSI_Control_BIO1/3(P_ref)
  [Qi_diesel] -> CSI_Control_BIO1/4(Q_ref)
  Gain17/1 -> Product3/1
  [Pi_bio] -> CSI_Control_BIO/3(P_ref)
  [Qi_bio] -> CSI_Control_BIO/4(Q_ref)
  [Q_ref] -> Gain20/1
  Gain20/1 -> Scope12/2
  MATLAB Function3/1(y) -> Scope22/1
  From37/1 -> MATLAB Function3/3(potencia)
  From38/1 -> MATLAB Function4/1(u)
  From40/1 -> MATLAB Function4/2(pref)
  From39/1 -> MATLAB Function4/3(qref)
  Power1/1 -> Goto75/1, MATLAB Function4/4(pm)
  Power1/2 -> Goto74/1, MATLAB Function4/5(qm)
  MATLAB Function4/1(y) -> Scope35/1
  MATLAB Function4/2(pam) -> Scope35/2
  Constant30/1 -> Diesel Generator2/2(Par de Carga)
  Transfer Fcn4/1 -> Goto24/1
  Sum13/1 -> PID Controller2/1
  From41/1 -> Gain21/1
  Gain21/1 -> Sum15/2
  PID Controller2/1 -> Diesel Generator2/1(in)
  Sum15/1 -> Goto23/1, Scope37/1, Sum13/2, Transfer Fcn4/1  "Output DC Voltage"
  Constant29/1 -> Sum13/1
  Diesel Generator2/2(Power) -> Sum15/1
  Diesel Generator2/3(caudal) -> Scope38/1
  Power3/1 -> MATLAB Function5/1(p)
  Power3/2 -> MATLAB Function5/2(q)
  MATLAB Function5/1(y) -> Scope39/1
  Power4/2 -> MATLAB Function6/2(q)
  Power4/1 -> MATLAB Function6/1(p)
  MATLAB Function6/1(y) -> Scope40/1
  From47/1 -> Power4/2
  Demux3/4 -> [Qi_diesel]
  Demux3/3 -> [Pi_Diesel]
  Demux3/2 -> [Qi_bio]
  Demux3/1 -> [Pi_bio]
  cdis4/1 -> [yest], Sum33/1, [x_hat], Signal Specification/1, Scope8/1, Sum17/2
  [V_vsi] -> Mux8/4
  MATLAB Function7/1(y) -> Demux19/1
  Sum17/1 -> Derivative4/1, MATLAB Function7/1(r), Scope48/1, adis10/1
  Mux7/1 -> To Workspace3/1, To Workspace15/1, [u_fs]
  MATLAB Function8/2(norm_rd) -> Sum41/1, Memory14/1, To Workspace1/1, Scope50/1
  Clock1/1 -> MATLAB Function8/3(tiempo)
  bdis5/1 -> Sum75/1
  Signal Specification/1 -> MATLAB Function8/1(y_hat)
  Demux19/2 -> Scope54/2
  [y_ma] -> Sum17/1
  [I3] -> Mux8/3
  [I2] -> Mux8/2
  [u_fs] -> bdis5/1
  Mux8/1 -> To Workspace6/1, To Workspace2/1, [y_ma]
  Derivative4/1 -> Scope139/1
  Signal Specification1/1 -> MATLAB Function8/2(y_m)
  adis7/1 -> Sum75/3
  From60/1 -> Signal Specification1/1
  Unit Delay6/1 -> cdis4/1, adis7/1
  adis10/1 -> Sum75/2
  Sum75/1 -> Unit Delay6/1
  [I1] -> Mux8/1
  Demux19/1 -> Scope54/1
  Demux19/3 -> Scope54/3
  Demux19/4 -> Scope54/4
  [u1] -> Mux7/1
  [u2] -> Mux7/2
  [u3] -> Mux7/3
  [y_ma] -> Scope8/2
  MATLAB Function8/1(rol) -> To Workspace/1, Scope9/1
  bdis9/1 -> Sum10/2
  bdis11/1 -> Sum23/2
  Unit Delay7/1 -> adis11/1, bdis15/1, Sum10/1
  adis12/1 -> Sum23/3
  bdis21/1 -> Sum19/1
  Sum31/1 -> Scope65/1
  [I2] -> bdis14/1, bdis9/1, bdis8/1
  [y_ma] -> Scope86/1
  [u_fs] -> bdis1/1
  [y_ma] -> Scope88/1
  adis11/1 -> Sum21/3
  Sum76/1 -> Unit Delay2/1
  bdis14/1 -> Sum31/2
  bdis12/1 -> Sum22/2
  Unit Delay10/1 -> bdis16/1, adis12/1, Sum22/1
  bdis3/1 -> Sum38/2
  Sum32/1 -> Scope66/1
  [I3] -> bdis13/1, bdis12/1, bdis11/1
  Unit Delay2/1 -> bdis21/1, adis2/1, Sum74/1
  bdis4/1 -> Sum71/2
  bdis2/1 -> Sum49/2
  [y_ma] -> Scope89/1
  Unit Delay1/1 -> bdis6/1, adis1/1, Sum38/1
  adis1/1 -> Sum49/3
  bdis10/1 -> Sum23/1
  [u_fs] -> bdis7/1
  bdis17/1 -> Sum76/1
  bdis18/1 -> Sum76/2
  [u_fs] -> bdis10/1
  bdis13/1 -> Sum32/2
  Sum21/1 -> Unit Delay7/1
  bdis6/1 -> Sum71/1
  bdis7/1 -> Sum21/1
  Sum19/1 -> Scope72/1
  bdis20/1 -> Sum19/2
  bdis1/1 -> Sum49/1
  bdis16/1 -> Sum32/1
  adis2/1 -> Sum76/3
  [V_vsi] -> bdis4/1, bdis3/1, bdis2/1
  bdis15/1 -> Sum31/1
  Sum49/1 -> Unit Delay1/1
  [I1] -> bdis20/1, bdis19/1, bdis18/1
  [y_ma] -> Scope87/1
  Sum22/1 -> cdis2/1
  bdis19/1 -> Sum74/2
  Sum74/1 -> cdis5/1
  Sum71/1 -> Scope67/1
  Sum23/1 -> Unit Delay10/1
  [u_fs] -> bdis17/1
  bdis8/1 -> Sum21/2
  cdis1/1 -> Demux7/1, Memory10/1, Sum36/1, Sum46/2, Scope86/2, Scope61/1
  Sum38/1 -> cdis3/1
  [x_hat_uio21] -> Sum67/1
  [y_ma] -> Sum67/2
  [x_hat_uio11] -> Sum70/1
  [y_ma] -> Sum70/2
  [x_hat_uio12] -> Sum72/1
  [y_ma] -> Sum72/2
  [x_hat_uio13] -> Sum73/1
  [y_ma] -> Sum73/2
  [druo3] -> Sum77/3
  [druo2] -> Sum77/2
  Sum77/1 -> Gain22/1
  [druo1] -> Sum77/1
  Gain22/1 -> Demux8/1, Abs/1, [uio1], Scope110/1
  Sum78/1 -> Gain23/1
  [druo3] -> Sum78/2
  [druo2] -> Sum78/1
  [druo4] -> Sum78/3
  [druo4] -> Sum79/3
  Sum79/1 -> Gain24/1
  [druo1] -> Sum79/2
  [druo3] -> Sum79/1
  [druo1] -> Sum80/3
  Sum80/1 -> Gain25/1
  [druo2] -> Sum80/2
  [druo4] -> Sum80/1
  Gain23/1 -> Demux16/1, Abs2/1, [uio2], Scope112/1
  Gain24/1 -> Demux15/1, Abs1/1, [uio3], Scope114/1
  MeasureNode_I1/1(Out) -> [I2], [i2]
  MeasureNode_I3/1(Out) -> [I3], [i3]
  Sum70/1 -> [druo1], Scope30/1
  Sum72/1 -> [druo2], Scope43/1
  Sum73/1 -> [druo3], Scope44/1
  Sum67/1 -> [druo4], Scope45/1
  Memory/1 -> Sum20/2
  Constant8/1 -> Switch/1
  MATLAB Function36/1(r) -> Sum53/2
  MATLAB Function36/2(c) -> [ruo1], Scope121/1, Memory1/1
  Switch/1 -> MATLAB Function36/2(ban)
  Sum53/1 -> Scope120/1
  Memory1/1 -> Switch/2
  Constant9/1 -> Switch/3
  Constant5/1 -> Sum53/1
  Memory2/1 -> Sum24/2
  Memory3/1 -> Sum25/2
  Memory4/1 -> Sum26/2
  Sum26/1 -> Product4/1, Scope46/1
  Constant6/1 -> Sum28/1
  Constant10/1 -> Switch1/3
  Switch1/1 -> MATLAB Function17/2(ban)
  MATLAB Function17/2(c) -> [ruo2], Scope49/1, Memory5/1
  Memory5/1 -> Switch1/2
  Sum28/1 -> Scope47/1
  Constant7/1 -> Switch1/1
  MATLAB Function17/1(r) -> Sum28/2
  Constant12/1 -> Sum29/1
  Constant22/1 -> Switch2/3
  Switch2/1 -> MATLAB Function18/2(ban)
  MATLAB Function18/2(c) -> [ruo4], Scope56/1, Memory6/1
  Memory6/1 -> Switch2/2
  Sum29/1 -> Scope55/1
  Constant21/1 -> Switch2/1
  MATLAB Function18/1(r) -> Sum29/2
  Memory7/1 -> Sum30/2
  [y_ma] -> Sum33/2
  Sum33/1 -> Sum30/1, Memory7/1
  Constant23/1 -> Sum34/1
  Constant27/1 -> Switch3/3
  Switch3/1 -> Scope75/1, MATLAB Function12/2(ban)
  MATLAB Function12/2(c) -> [rol], Scope69/1, Memory8/1
  Memory8/1 -> Switch3/2
  Sum34/1 -> Scope68/1
  Constant24/1 -> Switch3/1
  MATLAB Function12/1(r) -> Sum34/2
  Sum30/1 -> Abs5/1
  Constant28/1 -> Sum35/1
  Constant31/1 -> Switch4/1
  Sum24/1 -> To Workspace13/1, Demux11/1, MATLAB Function13/1(dr)
  Sum35/1 -> Scope51/1
  MATLAB Function13/1(r) -> Sum35/2
  Memory9/1 -> Switch4/2
  Switch4/1 -> MATLAB Function13/2(ban)
  MATLAB Function13/2(c) -> [ruo3], Scope57/1, Memory9/1
  Constant32/1 -> Switch4/3
  Clock2/1 -> MATLAB Function13/3(t)
  Memory10/1 -> Sum36/2
  Memory11/1 -> Sum37/2
  Memory12/1 -> Sum39/2
  Memory13/1 -> Sum40/2
  Abs1/1 -> Memory2/1, Sum24/1, Scope31/1
  Abs/1 -> Memory/1, Sum20/1, Scope25/1
  Abs2/1 -> Memory3/1, Sum25/1, Scope34/1
  Abs3/1 -> Memory4/1, Sum26/1
  Demux1/1 -> Scope77/1
  Demux1/2 -> Scope77/2
  Demux1/3 -> Scope77/3
  Demux1/4 -> Scope77/4
  Sum37/1 -> Demux1/1
  Demux2/1 -> Scope76/1
  Demux2/2 -> Scope76/2
  Demux2/4 -> Scope76/4
  Demux2/3 -> Scope76/3
  Sum36/1 -> Demux2/1
  Demux4/1 -> Scope78/1
  Demux4/2 -> Scope78/2
  Demux4/4 -> Scope78/4
  Demux4/3 -> Scope78/3
  Sum39/1 -> Demux4/1
  Demux9/1 -> Scope79/1
  Demux9/2 -> Scope79/2
  Demux9/4 -> Scope79/4
  Demux9/3 -> Scope79/3
  Sum40/1 -> Demux9/1
  Demux10/1 -> Scope119/1, Scope80/1
  Demux10/2 -> Scope122/1, Scope80/2
  Demux10/4 -> Scope142/1, Scope80/4
  Demux10/3 -> Scope141/1, Scope80/3
  Demux11/1 -> Scope81/1
  Demux11/2 -> Scope81/2
  Demux11/4 -> Scope81/4
  Demux11/3 -> Scope81/3
  Demux12/1 -> Scope82/1
  Demux12/2 -> Scope82/2
  Demux12/4 -> Scope82/4
  Demux12/3 -> Scope82/3
  Demux13/1 -> Scope83/1
  Demux13/2 -> Scope83/2
  Demux13/4 -> Scope83/4
  Demux13/3 -> Scope83/3
  Demux14/3 -> Scope33/3
  Demux14/4 -> Delay/1, Scope33/4
  Demux14/2 -> Scope33/2
  Demux14/1 -> Scope33/1
  Abs5/1 -> Demux14/1, MATLAB Function12/1(dr)
  Memory14/1 -> Sum41/2
  Sum41/1 -> Abs4/1
  Abs4/1 -> Scope36/1
  [x_hat_uio3] -> MATLAB Function39/3(x_hat3)
  [x_hat_uio1] -> MATLAB Function38/1(x_hat1)
  [x_hat_uio4] -> MATLAB Function39/4(x_hat4)
  [rol] -> MATLAB Function39/6(rol)
  [x_hat_uio1] -> MATLAB Function39/1(x_hat1)
  [rol] -> MATLAB Function34/6(rol)
  [ruo1] -> MATLAB Function38/5(ruo1)
  [x_hat_uio4] -> MATLAB Function34/4(x_hat4)
  [x_hat_uio1] -> MATLAB Function34/1(x_hat1)
  [x_hat_uio4] -> MATLAB Function38/4(x_hat4)
  [ruo3] -> MATLAB Function39/5(ruo1)
  MATLAB Function34/1(v1) -> [ca2], Sum18/1, Scope53/1
  [x_hat_uio3] -> MATLAB Function34/3(x_hat3)
  [ruo2] -> MATLAB Function34/5(ruo1)
  [x_hat_uio2] -> MATLAB Function34/2(x_hat2)
  [rol] -> MATLAB Function38/6(rol)
  MATLAB Function39/1(v1) -> [ca3], Sum42/1, Scope58/1
  [x_hat_uio2] -> MATLAB Function38/2(x_hat2)
  [x_hat_uio2] -> MATLAB Function39/2(x_hat2)
  [x_hat_uio3] -> MATLAB Function38/3(x_hat3)
  [x_hat_uio21] -> Sum59/1
  [x_hat_uio11] -> Sum58/1
  [x_hat_uio12] -> Sum58/2
  Gain27/1 -> Scope135/1, Scope62/1, [x_hat_uio4]
  [x_hat_uio21] -> Sum60/3
  [x_hat_uio21] -> Sum61/2
  Sum58/1 -> Gain28/1
  [x_hat_uio13] -> Sum59/3
  Gain26/1 -> Scope42/1, Scope60/1, [x_hat_uio3]
  Sum60/1 -> Gain26/1
  [x_hat_uio12] -> Sum61/3
  Gain28/1 -> Scope138/1, [x_hat_uio1]
  [x_hat_uio13] -> Sum58/3
  [x_hat_uio11] -> Sum60/1
  [x_hat_uio13] -> Sum60/2
  Gain29/1 -> Scope59/1, Scope41/1, [x_hat_uio2]
  Sum61/1 -> Gain27/1
  [x_hat_uio11] -> Sum61/1
  [x_hat_uio12] -> Sum59/2
  Sum59/1 -> Gain29/1
  [ruo4] -> MATLAB Function1/5(ruo1)
  [x_hat_uio3] -> MATLAB Function1/3(x_hat3)
  [x_hat_uio1] -> MATLAB Function1/1(x_hat1)
  [x_hat_uio2] -> MATLAB Function1/2(x_hat2)
  [rol] -> MATLAB Function1/6(rol)
  [x_hat_uio4] -> MATLAB Function1/4(x_hat4)
  MeasureNode_I2/2(Out1) -> [a1]
  MeasureNode_I1/2(Out1) -> [a2]
  MeasureNode_I3/2(Out1) -> [a3]
  [a1] -> Sum16/2, Scope109/2
  [a2] -> Sum18/2, Scope53/2
  [a4] -> Sum27/2, Scope52/2
  [a3] -> Sum42/2, Scope58/2
  [x_hat] -> Scope138/2
  [y_ma] -> Scope138/3
  [y_ma] -> Scope59/3
  [x_hat] -> Scope59/2
  [y_ma] -> Scope60/3
  [x_hat] -> Scope60/2
  [y_ma] -> Scope62/3
  [x_hat] -> Scope62/2
  Sum16/1 -> Abs6/1
  Abs6/1 -> [e1], Scope64/1
  Sum18/1 -> Abs7/1
  Abs7/1 -> [e2], Scope70/1
  Sum27/1 -> Abs8/1
  Abs8/1 -> [e4], Scope71/1
  MATLAB Function1/1(v1) -> [ca4], Sum27/1, Scope52/1
  Sum42/1 -> Abs9/1
  Abs9/1 -> [e3], Scope73/1
  MeasureNode_I4/2(Out1) -> [a4]
  MeasureNode_I4/1(Out) -> [Vload], [V_vsi]
  MeasureNode_I5/1(Out) -> Goto61/1
  MeasureNode_I5/2(Out1) -> Goto62/1
  [rol] -> Scope84/1
  [ruo4] -> Scope84/5
  [ruo3] -> Scope84/4
  [ruo1] -> Scope84/2
  [ruo2] -> Scope84/3
  Delay/1 -> MATLAB Function12/3(dr1)
  MATLAB Function38/1(v1) -> [ca1], Sum16/1, Scope109/1
  [ca4] -> Scope85/4
  [ca3] -> Scope85/3
  [ca2] -> Scope85/2
  [ca1] -> Scope85/1
  [e4] -> Scope63/4
  [e3] -> Scope63/3
  [e2] -> Scope63/2
  [e1] -> Scope63/1
  CSI_Control_BIO/1(D) -> Scope13/1, Gain15/1
  CSI_Control_BIO1/1(D) -> Gain16/1, Scope20/1
  Sum43/1 -> Scope91/1
  From154/1 -> Scope95/2, Sum43/2
  Constant15/1 -> LinearProg2/1(P_load), [P_ref]
  Constant17/1 -> [Q_ref], LinearProg3/1(Q_load)
  Constant33/1 -> MeasureNode_I2/2(in1)
  Constant34/1 -> MeasureNode_I1/2(in1)
  Constant35/1 -> MeasureNode_I3/2(in1)
  Derivative1/1 -> Gain30/1
  Gain30/1 -> Sum45/1
  Sum45/1 -> Sum44/1
  Sine Wave6/1 -> Derivative1/1  "ref voltage"
  [i3] -> Sum45/2
  [i3m] -> Sum44/2
  Sine Wave4/1 -> Scope95/1, Sum43/1
  Constant36/1 -> MeasureNode_I4/2(in1)
  MeasureNode_I2/1(Out) -> [i1], [I1]
  [Qo_diesel] -> MATLAB Function2/2(q)
  [Po_diesel] -> MATLAB Function2/3(p)
  From161/1 -> Display/1, Scope92/1, Sum11/1  "Pdiesel"
  From165/1 -> Sum12/1, Display6/1, Scope93/1  "Qdiesel"
  From163/1 -> Sum11/2, Display1/1, Scope92/2  "Pbio"
  From162/1 -> Display2/1, Sum11/3, Scope92/3  "Pren"
  From164/1 -> Sum12/3, Display7/1, Scope93/2  "Qbio"
  From160/1 -> Sum12/2, Display8/1, Scope93/3  "Qren"
  Sum11/1 -> Display3/1, Scope92/4  "Ptotal"
  Sum12/1 -> Display9/1, Scope93/4  "Qtotal"
  Power/1 -> Display4/1, Scope11/1, Scope10/1
  [Qi_diesel] -> Display10/1, Scope17/2
  Sine Wave/1 -> Transfer Fcn5/1, Transfer Fcn2/1
  Transfer Fcn2/1 -> Scope94/1
  Transfer Fcn5/1 -> Scope96/1
  [Po_bio] -> Scope99/1
  [Qo_diesel] -> Scope100/1
  [Qo_bio] -> Scope98/1
  [Po_diesel] -> Scope101/1
  Mux3/1 -> Scope32/1, Demux6/1, MPC Controller/2
  Demux6/1 -> Scope99/2
  Demux6/2 -> Scope98/2
  Demux6/3 -> Scope101/2
  Demux6/4 -> Scope100/2
  Constant25/1 -> Product/1
  Constant4/1 -> Product3/2
  Clock/1 -> MATLAB Function12/4(t)
  Step13/1 -> Product2/2
  Sum25/1 -> Product2/1
  Product2/1 -> To Workspace12/1, MATLAB Function17/1(dr), Demux12/1
  Step14/1 -> Product4/2
  Product4/1 -> To Workspace14/1, MATLAB Function18/1(dr), Demux13/1
  Mux26/1 -> Scope74/1
  From177/1 -> Scope90/2
  From169/1 -> Mux26/2
  Mux27/1 -> Scope90/1
  From176/1 -> Scope97/2
  From171/1 -> Mux27/1
  Mux28/1 -> Scope97/1
  From167/1 -> Mux28/2
  From174/1 -> Scope74/2
  [Vlreal] -> Scope102/1
  From172/1 -> Mux28/1
  [V_vsi] -> Scope102/2
  From170/1 -> Mux26/1
  From168/1 -> Mux27/2
  From181/1 -> Scope103/1
  From185/1 -> Scope107/1
  From188/1 -> Scope106/2
  From189/1 -> Scope107/2
  From182/1 -> Scope104/2
  From183/1 -> Scope104/1
  From186/1 -> Scope106/1
  From184/1 -> Scope105/1
  From187/1 -> Scope105/2
  Demux5/4 -> Goto82/1
  Demux5/3 -> Goto81/1
  Demux5/1 -> Goto79/1
  Demux5/2 -> Goto80/1
  Function Fitting Neural Network/1(Output) -> Demux5/1
  From191/1 -> Mux1/3
  From190/1 -> Mux1/2
  From192/1 -> Mux1/1
  Mux1/1 -> Delay1/1
  Mux/1 -> Function Fitting Neural Network/1(Input)
  Delay1/1 -> Mux/2
  Delay2/1 -> Mux9/1
  Mux2/1 -> To Workspace4/1, State-Space/1
  State-Space/1 -> To Workspace5/1, Demux/1
  From/1 -> Scope/2
  From7/1 -> Scope3/2
  From8/1 -> Scope7/2
  Demux/1 -> Goto/1
  From24/1 -> Scope7/1
  From6/1 -> Scope1/2
  Demux/4 -> Goto22/1
  Demux/3 -> Goto16/1
  From33/1 -> Mux2/3
  From15/1 -> Scope1/1
  Demux/2 -> Goto15/1
  From25/1 -> Scope3/1
  From30/1 -> Mux2/2
  From14/1 -> Scope/1
  From9/1 -> Mux2/1
  Delay3/1 -> Mux9/2
  Delay4/1 -> Mux9/3
  Delay5/1 -> Mux9/4
  Delay6/1 -> Mux9/5
  Delay7/1 -> Mux9/6
  Delay8/1 -> Mux9/7
  Delay9/1 -> Mux9/8
  Delay10/1 -> Mux9/9
  Delay11/1 -> Mux9/10
  From193/1 -> Delay12/1, Delay11/1, Delay10/1, Delay9/1, Delay8/1, Delay7/1, Delay6/1, Delay5/1, Delay4/1, Delay3/1, Delay2/1
  Delay12/1 -> Mux9/11
  From194/1 -> Delay15/1, Delay14/1, Delay13/1, Delay23/1, Delay22/1, Delay21/1, Delay20/1, Delay19/1, Delay18/1, Delay17/1, Delay16/1
  Delay15/1 -> Mux10/11
  Delay19/1 -> Mux10/4
  Delay23/1 -> Mux10/8
  Delay17/1 -> Mux10/2
  Delay14/1 -> Mux10/10
  Delay13/1 -> Mux10/9
  Delay16/1 -> Mux10/1
  Delay22/1 -> Mux10/7
  Delay21/1 -> Mux10/6
  Delay18/1 -> Mux10/3
  Delay20/1 -> Mux10/5
  From195/1 -> Delay26/1, Delay25/1, Delay24/1, Delay45/1, Delay44/1, Delay43/1, Delay42/1, Delay41/1, Delay40/1, Delay39/1, Delay34/1
  Delay26/1 -> Mux12/11
  Delay41/1 -> Mux12/4
  Delay37/1 -> Mux11/7
  Delay28/1 -> Mux11/10
  From196/1 -> Delay29/1, Delay28/1, Delay27/1, Delay38/1, Delay37/1, Delay36/1, Delay35/1, Delay33/1, Delay32/1, Delay31/1, Delay30/1
  Delay29/1 -> Mux11/11
  Delay32/1 -> Mux11/3
  Delay35/1 -> Mux11/5
  Delay38/1 -> Mux11/8
  Delay36/1 -> Mux11/6
  Delay33/1 -> Mux11/4
  Delay45/1 -> Mux12/8
  Delay31/1 -> Mux11/2
  Delay39/1 -> Mux12/2
  Delay25/1 -> Mux12/10
  Delay24/1 -> Mux12/9
  Delay30/1 -> Mux11/1
  Delay27/1 -> Mux11/9
  Delay34/1 -> Mux12/1
  Delay44/1 -> Mux12/7
  Delay43/1 -> Mux12/6
  Delay40/1 -> Mux12/3
  Delay42/1 -> Mux12/5
  Mux9/1 -> Goto83/1
  Mux10/1 -> Goto84/1
  Mux12/1 -> Goto85/1
  Mux11/1 -> Goto86/1
  Mux13/1 -> Mux/1
  From197/1 -> Mux13/1
  From198/1 -> Mux13/2
  From199/1 -> Mux13/3
  From200/1 -> Mux13/4
  From203/1 -> Mux15/1
  From202/1 -> Mux15/3
  From201/1 -> Mux15/2
  Mux14/1 -> Function Fitting Neural Network1/1(Input)
  Mux16/1 -> Function Fitting Neural Network2/1(Input)
  Mux17/1 -> Function Fitting Neural Network3/1(Input)
  Mux18/1 -> Function Fitting Neural Network4/1(Input)
  Function Fitting Neural Network2/1(Output) -> Goto88/1
  Function Fitting Neural Network1/1(Output) -> Goto87/1
  Function Fitting Neural Network3/1(Output) -> Goto89/1
  Function Fitting Neural Network4/1(Output) -> Goto90/1
  Mux21/1 -> Goto93/1
  Delay84/1 -> Mux21/7
  Delay82/1 -> Mux21/5
  Delay83/1 -> Mux21/6
  Delay73/1 -> Mux21/1
  Delay85/1 -> Mux21/8
  Delay78/1 -> Mux21/2
  Delay81/1 -> Mux21/4
  From206/1 -> Delay64/1, Delay63/1, Delay62/1, Delay85/1, Delay84/1, Delay83/1, Delay82/1, Delay81/1, Delay80/1, Delay78/1, Delay73/1
  Delay80/1 -> Mux21/3
  Delay62/1 -> Mux21/9
  Delay63/1 -> Mux21/10
  Delay64/1 -> Mux21/11
  From208/1 -> Mux14/1
  From209/1 -> Mux16/1
  From210/1 -> Mux17/1
  From211/1 -> Mux18/1
  From214/1 -> Scope111/1
  From216/1 -> Scope113/1
  From217/1 -> Scope111/2
  From212/1 -> Scope108/2
  From215/1 -> Scope115/1
  From218/1 -> Scope113/2
  From213/1 -> Scope108/1
  From219/1 -> Scope115/2
  Delay92/1 -> Mux23/11
  Delay46/1 -> Mux23/9
  From220/1 -> Delay93/1, Delay92/1, Delay91/1, Delay46/1, Delay100/1, Delay99/1, Delay98/1, Delay97/1, Delay96/1, Delay95/1, Delay94/1
  Delay91/1 -> Mux23/10
  Delay93/1 -> Mux23/1
  Delay96/1 -> Mux23/4
  Delay97/1 -> Mux23/5
  Delay94/1 -> Mux23/2
  Delay100/1 -> Mux23/8
  Delay95/1 -> Mux23/3
  Delay99/1 -> Mux23/7
  Mux23/1 -> Goto95/1
  Delay98/1 -> Mux23/6
  Mux24/1 -> Goto96/1
  Delay105/1 -> Mux24/1
  Delay110/1 -> Mux24/6
  Delay109/1 -> Mux24/5
  Delay101/1 -> Mux24/8
  Delay111/1 -> Mux24/7
  Delay108/1 -> Mux24/4
  Delay106/1 -> Mux24/2
  Delay103/1 -> Mux24/10
  Delay107/1 -> Mux24/3
  From221/1 -> Delay105/1, Delay104/1, Delay103/1, Delay102/1, Delay101/1, Delay111/1, Delay110/1, Delay109/1, Delay108/1, Delay107/1, Delay106/1
  Delay104/1 -> Mux24/11
  Delay102/1 -> Mux24/9
  Mux25/1 -> Goto97/1
  Delay116/1 -> Mux25/1
  Delay121/1 -> Mux25/6
  Delay120/1 -> Mux25/5
  Delay112/1 -> Mux25/8
  Delay122/1 -> Mux25/7
  Delay119/1 -> Mux25/4
  Delay117/1 -> Mux25/2
  Delay114/1 -> Mux25/10
  Delay118/1 -> Mux25/3
  From222/1 -> Delay116/1, Delay115/1, Delay114/1, Delay113/1, Delay112/1, Delay122/1, Delay121/1, Delay120/1, Delay119/1, Delay118/1, Delay117/1
  Delay115/1 -> Mux25/11
  Delay113/1 -> Mux25/9
  MATLAB Function/1(yu) -> Scope117/2
  MATLAB Function/2(yl) -> Scope117/3
  Demux7/2 -> Scope117/1, MATLAB Function/1(u)
  Delay51/1 -> Mux19/2
  Delay49/1 -> Mux19/11
  Delay56/1 -> Mux19/7
  Mux19/1 -> Goto91/1
  Delay52/1 -> Mux19/3
  Delay48/1 -> Mux19/10
  From204/1 -> Delay49/1, Delay48/1, Delay47/1, Delay57/1, Delay56/1, Delay55/1, Delay54/1, Delay53/1, Delay52/1, Delay51/1, Delay50/1
  Delay47/1 -> Mux19/9
  Delay50/1 -> Mux19/1
  Delay54/1 -> Mux19/5
  Delay53/1 -> Mux19/4
  Delay57/1 -> Mux19/8
  Delay55/1 -> Mux19/6
  Delay65/1 -> Mux20/2
  Delay60/1 -> Mux20/11
  Delay70/1 -> Mux20/7
  Mux20/1 -> Goto92/1
  Delay66/1 -> Mux20/3
  Delay59/1 -> Mux20/10
  From205/1 -> Delay60/1, Delay59/1, Delay58/1, Delay71/1, Delay70/1, Delay69/1, Delay68/1, Delay67/1, Delay66/1, Delay65/1, Delay61/1
  Delay58/1 -> Mux20/9
  Delay61/1 -> Mux20/1
  Delay68/1 -> Mux20/5
  Delay67/1 -> Mux20/4
  Delay71/1 -> Mux20/8
  Delay69/1 -> Mux20/6
  Delay77/1 -> Mux22/2
  Delay75/1 -> Mux22/11
  Delay89/1 -> Mux22/7
  Mux22/1 -> Goto94/1
  Delay79/1 -> Mux22/3
  Delay74/1 -> Mux22/10
  From207/1 -> Delay75/1, Delay74/1, Delay72/1, Delay90/1, Delay89/1, Delay88/1, Delay87/1, Delay86/1, Delay79/1, Delay77/1, Delay76/1
  Delay72/1 -> Mux22/9
  Delay76/1 -> Mux22/1
  Delay87/1 -> Mux22/5
  Delay86/1 -> Mux22/4
  Delay90/1 -> Mux22/8
  Delay88/1 -> Mux22/6
  Mux15/1 -> Mux14/2, Mux16/2, Mux18/2, Mux17/2
  Constant19/1 -> LinearProg3/5(QdMax)
  Constant14/1 -> LinearProg3/6(QbMax)
  Constant13/1 -> LinearProg3/7(Q_e_alt_min)
  Constant16/1 -> LinearProg2/5(PdMax)
  Constant20/1 -> LinearProg2/6(PbMax)
  Constant18/1 -> LinearProg2/7(P_e_alt_min)
  Demux15/3 -> To Workspace8/1
  Demux16/2 -> To Workspace9/1
  Demux17/4 -> To Workspace10/1
  Gain25/1 -> Demux17/1, [uio4], Scope118/1, Abs3/1
  Sum20/1 -> Demux10/1, To Workspace11/1, MATLAB Function36/1(dr), Umbral adaptativo17/2(u)
  Demux8/1 -> To Workspace7/1
  Constant38/1 -> Umbral adaptativo1/1(const)
  Demux18/1 -> MATLAB Function10/1(u1)
  Clock4/1 -> MATLAB Function10/3(t)
  Umbral adaptativo1/1(Out1) -> MATLAB Function10/2(u2)
  MATLAB Function10/2(y2) -> Scope123/2
  MATLAB Function10/1(y1) -> Scope123/1
  From225/1 -> Demux18/1
  MATLAB Function11/2(y2) -> Scope116/2
  MATLAB Function11/1(y1) -> Scope116/1
  Clock5/1 -> MATLAB Function11/3(t)
  Umbral adaptativo2/1(Out1) -> MATLAB Function11/2(u2)
  From224/1 -> Umbral adaptativo4/2(u), Umbral adaptativo3/2(u), Umbral adaptativo2/2(u), Umbral adaptativo1/2(u)
  Constant39/1 -> Umbral adaptativo2/1(const)
  Constant40/1 -> Umbral adaptativo3/1(const)
  Constant41/1 -> Umbral adaptativo4/1(const)
  Demux18/2 -> MATLAB Function11/1(u1)
  Clock6/1 -> MATLAB Function14/3(t)
  MATLAB Function14/1(y1) -> Scope124/1
  MATLAB Function14/2(y2) -> Scope124/2
  Umbral adaptativo3/1(Out1) -> MATLAB Function14/2(u2)
  Demux18/3 -> MATLAB Function14/1(u1)
  Clock7/1 -> MATLAB Function15/3(t)
  MATLAB Function15/1(y1) -> Scope125/1
  MATLAB Function15/2(y2) -> Scope125/2
  Umbral adaptativo4/1(Out1) -> MATLAB Function15/2(u2)
  Demux18/4 -> MATLAB Function15/1(u1)
  MATLAB Function16/2(y2) -> Scope127/2
  MATLAB Function16/1(y1) -> Scope127/1
  Constant42/1 -> Umbral adaptativo5/1(const)
  Demux20/4 -> MATLAB Function21/1(u1)
  Clock9/1 -> MATLAB Function19/3(t)
  MATLAB Function19/1(y1) -> Scope126/1
  MATLAB Function21/2(y2) -> Scope129/2
  MATLAB Function21/1(y1) -> Scope129/1
  Clock11/1 -> MATLAB Function21/3(t)
  From226/1 -> Umbral adaptativo8/2(u), Umbral adaptativo7/2(u), Umbral adaptativo6/2(u), Umbral adaptativo5/2(u)
  Demux20/1 -> MATLAB Function16/1(u1)
  Umbral adaptativo5/1(Out1) -> MATLAB Function16/2(u2)
  Umbral adaptativo7/1(Out1) -> MATLAB Function20/2(u2)
  Clock10/1 -> MATLAB Function20/3(t)
  MATLAB Function20/2(y2) -> Scope128/2
  Constant45/1 -> Umbral adaptativo8/1(const)
  MATLAB Function20/1(y1) -> Scope128/1
  Clock8/1 -> MATLAB Function16/3(t)
  Demux20/2 -> MATLAB Function19/1(u1)
  Umbral adaptativo8/1(Out1) -> MATLAB Function21/2(u2)
  Demux20/3 -> MATLAB Function20/1(u1)
  From227/1 -> Demux20/1
  Constant43/1 -> Umbral adaptativo6/1(const)
  Constant44/1 -> Umbral adaptativo7/1(const)
  MATLAB Function19/2(y2) -> Scope126/2
  Umbral adaptativo6/1(Out1) -> MATLAB Function19/2(u2)
  MATLAB Function22/1(y1) -> Scope131/1
  Umbral adaptativo14/1(Out1) -> MATLAB Function27/2(u2)
  Constant51/1 -> Umbral adaptativo14/1(const)
  From231/1 -> Demux22/1
  Demux22/3 -> MATLAB Function28/1(u1)
  Constant46/1 -> Umbral adaptativo9/1(const)
  Constant53/1 -> Umbral adaptativo16/1(const)
  MATLAB Function28/2(y2) -> Scope137/2
  Constant52/1 -> Umbral adaptativo15/1(const)
  Clock18/1 -> MATLAB Function26/3(t)
  MATLAB Function22/2(y2) -> Scope131/2
  Clock12/1 -> MATLAB Function28/3(t)
  Umbral adaptativo13/1(Out1) -> MATLAB Function26/2(u2)
  Demux22/1 -> MATLAB Function26/1(u1)
  MATLAB Function28/1(y1) -> Scope137/1
  Umbral adaptativo16/1(Out1) -> MATLAB Function29/2(u2)
  From230/1 -> Umbral adaptativo16/2(u), Umbral adaptativo15/2(u), Umbral adaptativo14/2(u), Umbral adaptativo13/2(u)
  MATLAB Function27/1(y1) -> Scope134/1
  MATLAB Function27/2(y2) -> Scope134/2
  MATLAB Function29/2(y2) -> Scope140/2
  Clock19/1 -> MATLAB Function27/3(t)
  MATLAB Function26/1(y1) -> Scope136/1
  Demux22/2 -> MATLAB Function27/1(u1)
  Demux21/4 -> MATLAB Function25/1(u1)
  Clock15/1 -> MATLAB Function23/3(t)
  MATLAB Function23/1(y1) -> Scope130/1
  MATLAB Function25/2(y2) -> Scope133/2
  MATLAB Function25/1(y1) -> Scope133/1
  Demux22/4 -> MATLAB Function29/1(u1)
  Clock17/1 -> MATLAB Function25/3(t)
  From228/1 -> Umbral adaptativo12/2(u), Umbral adaptativo11/2(u), Umbral adaptativo10/2(u), Umbral adaptativo9/2(u)
  Demux21/1 -> MATLAB Function22/1(u1)
  Umbral adaptativo9/1(Out1) -> MATLAB Function22/2(u2)
  Umbral adaptativo11/1(Out1) -> MATLAB Function24/2(u2)
  Clock13/1 -> MATLAB Function29/3(t)
  Clock16/1 -> MATLAB Function24/3(t)
  MATLAB Function24/2(y2) -> Scope132/2
  Constant49/1 -> Umbral adaptativo12/1(const)
  MATLAB Function24/1(y1) -> Scope132/1
  MATLAB Function29/1(y1) -> Scope140/1
  Clock14/1 -> MATLAB Function22/3(t)
  Demux21/2 -> MATLAB Function23/1(u1)
  Umbral adaptativo12/1(Out1) -> MATLAB Function25/2(u2)
  Demux21/3 -> MATLAB Function24/1(u1)
  Constant50/1 -> Umbral adaptativo13/1(const)
  From229/1 -> Demux21/1
  Constant47/1 -> Umbral adaptativo10/1(const)
  Constant48/1 -> Umbral adaptativo11/1(const)
  MATLAB Function23/2(y2) -> Scope130/2
  Umbral adaptativo15/1(Out1) -> MATLAB Function28/2(u2)
  MATLAB Function26/2(y2) -> Scope136/2
  Umbral adaptativo10/1(Out1) -> MATLAB Function23/2(u2)
  Constant37/1 -> Umbral adaptativo17/1(const)
  Umbral adaptativo17/1(th1) -> Scope119/2
  Umbral adaptativo17/2(th2) -> Scope122/2
  Umbral adaptativo17/3(th3) -> Scope141/2
  Umbral adaptativo17/4(th4) -> Scope142/2
  [I1] -> Scope143/1
  [I3] -> Scope145/1
  [I2] -> Scope144/1
  Demux24/1 -> Scope143/2
  [yest] -> Demux24/1
  [V_vsi] -> Scope146/1
  Demux24/3 -> Scope145/2
  Demux24/4 -> Scope146/2
  Demux24/2 -> Scope144/2
  Demux26/3 -> Scope153/2
  Demux26/2 -> Scope152/2
  [I2] -> Scope152/1
  [I1] -> Scope151/1
  [I3] -> Scope153/1
  Demux26/1 -> Scope151/2
  [V_vsi] -> Scope154/1
  Demux26/4 -> Scope154/2
  [x_hat_uio11] -> Demux26/1
  Demux29/2 -> Scope164/2
  [I1] -> Scope163/1
  Demux29/3 -> Scope165/2
  [I2] -> Scope164/1
  Demux29/4 -> Scope166/2
  Demux29/1 -> Scope163/2
  [I3] -> Scope165/1
  [x_hat_uio12] -> Demux29/1
  [V_vsi] -> Scope166/1
  [x_hat_uio13] -> Demux28/1
  Demux28/4 -> Scope162/2
  [I3] -> Scope161/1
  Demux28/3 -> Scope161/2
  [I2] -> Scope160/1
  [V_vsi] -> Scope162/1
  Demux28/1 -> Scope159/2
  Demux28/2 -> Scope160/2
  [I1] -> Scope159/1
  [x_hat_uio21] -> Demux27/1
  Demux27/4 -> Scope158/2
  Demux27/3 -> Scope157/2
  [I2] -> Scope156/1
  [I3] -> Scope157/1
  Demux27/2 -> Scope156/2
  [V_vsi] -> Scope158/1
  [I1] -> Scope155/1
  Demux27/1 -> Scope155/2
  Sum10/1 -> cdis1/1
  Discrete State-Space/1 -> [x_hat_uio11], Sum46/1
  Sum46/1 -> Scope147/1
  Mux29/1 -> Discrete State-Space/1
  [u_fs] -> Mux29/1
  [I2] -> Mux29/2
  [I1] -> Mux30/2
  Sum47/1 -> Scope148/1
  Mux30/1 -> Discrete State-Space1/1
  cdis5/1 -> Sum47/2, Memory13/1, Sum40/1, Scope89/2
  Discrete State-Space1/1 -> [x_hat_uio21], Sum47/1
  [u_fs] -> Mux30/1
  [I3] -> Mux31/2
  Sum48/1 -> Scope149/1
  Mux31/1 -> Discrete State-Space2/1
  cdis2/1 -> Sum48/2, Memory11/1, Sum37/1, Scope87/2
  Discrete State-Space2/1 -> [x_hat_uio12], Sum48/1
  [u_fs] -> Mux31/1
  [V_vsi] -> Mux32/2
  Sum50/1 -> Scope150/1
  Mux32/1 -> Discrete State-Space3/1
  cdis3/1 -> Sum50/2, Memory12/1, Sum39/1, Scope88/2
  Discrete State-Space3/1 -> [x_hat_uio13], Sum50/1
  [u_fs] -> Mux32/1
  [I1r] -> Scope167/1
  [I1] -> Scope167/2
  [I2r] -> Scope168/1
  [I2] -> Scope168/2
